simulink model "mechanical"  (R2019b)
settings: Solver=VariableStepAuto  StartTime=0.0  StopTime=10.0  RelTol=1e-3
undefined symbols (not defined in the file): B_hs, B_ks, beta, Cp, Cv, F_L, Fc, K_hs, K_ks, M, M_L, P_0, S_0, S_A, S_B, x0
libraries: simulink x2
settings Model: Creator=artof  LastModifiedBy=artof

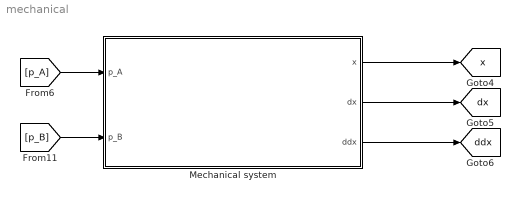
== system mechanical ==
  Mechanical system : Subsystem
  tag scope: ddx=global, dx=global, x=global
  wires:
  [p_A] -> Mechanical system/1(p_A)
  Mechanical system/1(x) -> [x]
  Mechanical system/2(dx) -> [dx]
  Mechanical system/3(ddx) -> [ddx]
  [p_B] -> Mechanical system/2(p_B)

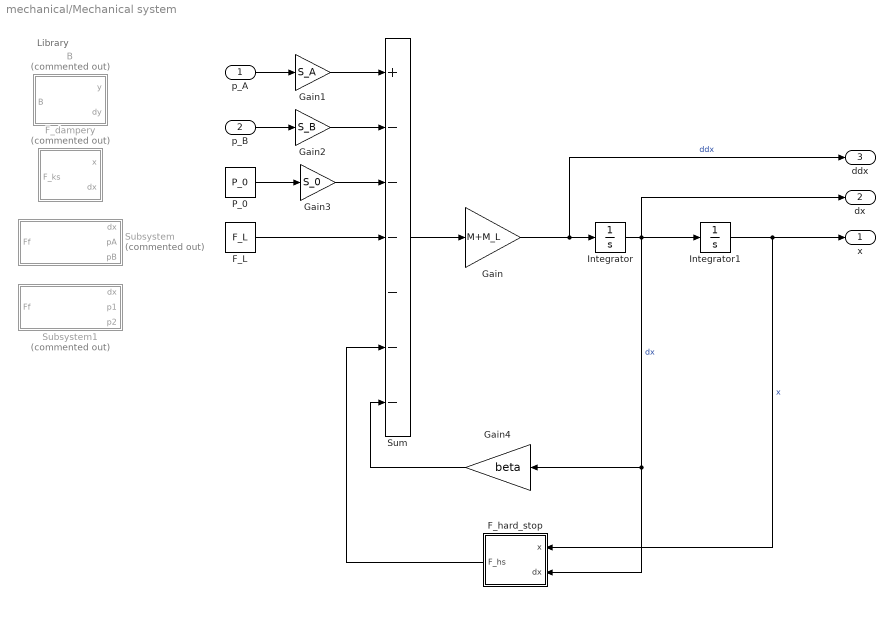
== system mechanical/Mechanical system ==
  note: Library
  p_A : Inport
  p_B : Inport  Port=2
  B : MATLAB Function  Commented=on  TreatAsAtomicUnit=on
  F_L : Constant  Value=F_L
  F_dampery : Subsystem  Commented=on
  F_hard_stop : Subsystem
  Gain : Gain  Gain=M+M_L
  Gain1 : Gain  Gain=S_A
  Gain2 : Gain  Gain=S_B
  Gain3 : Gain  Gain=S_0
  Gain4 : Gain  Gain=beta
  Integrator : Integrator
  Integrator1 : Integrator  InitialCondition=x0
  P_0 : Constant  Value=P_0
  Subsystem : Subsystem  Commented=on
  Subsystem1 : Subsystem  Commented=on
  Sum : Sum  Inputs=+------
  x : Outport
  dx : Outport  Port=2
  ddx : Outport  Port=3
  wires:
  p_A/1 -> Gain1/1
  Gain/1 -> ddx/1, Integrator/1  "ddx"
  Sum/1 -> Gain/1
  F_L/1 -> Sum/4
  P_0/1 -> Gain3/1
  Gain3/1 -> Sum/3
  Integrator/1 -> dx/1, F_hard_stop/2(dx), Gain4/1, Integrator1/1  "dx"
  Integrator1/1 -> x/1, F_hard_stop/1(x)  "x"
  p_B/1 -> Gain2/1
  Gain2/1 -> Sum/2
  F_hard_stop/1(F_hs) -> Sum/6
  Gain1/1 -> Sum/1
  Gain4/1 -> Sum/7

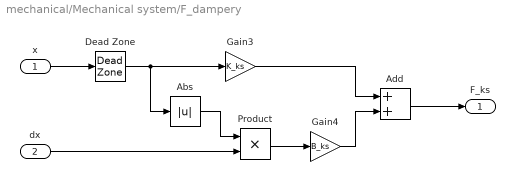
== system mechanical/Mechanical system/F_dampery ==
  x : Inport
  dx : Inport  Port=2
  Abs : Abs
  Add : Sum
  Dead Zone : DeadZone  LowerValue=0.02  UpperValue=0.180  SaturateOnIntegerOverflow=on
  Gain3 : Gain  Gain=K_ks
  Gain4 : Gain  Gain=B_ks
  Product : Product
  F_ks : Outport
  wires:
  Gain4/1 -> Add/2
  dx/1 -> Product/2
  Add/1 -> F_ks/1
  x/1 -> Dead Zone/1
  Gain3/1 -> Add/1
  Abs/1 -> Product/1
  Dead Zone/1 -> Abs/1, Gain3/1
  Product/1 -> Gain4/1

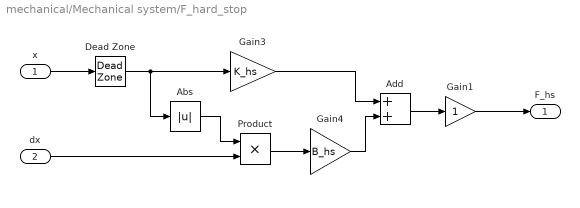
== system mechanical/Mechanical system/F_hard_stop ==
  x : Inport
  dx : Inport  Port=2
  Abs : Abs
  Add : Sum
  Dead Zone : DeadZone  LowerValue=0  UpperValue=L  SaturateOnIntegerOverflow=on
  Gain1 : Gain
  Gain3 : Gain  Gain=K_hs
  Gain4 : Gain  Gain=B_hs
  Product : Product
  F_hs : Outport
  wires:
  Product/1 -> Gain4/1
  Dead Zone/1 -> Gain3/1, Abs/1
  Abs/1 -> Product/1
  Gain3/1 -> Add/1
  x/1 -> Dead Zone/1
  Add/1 -> Gain1/1
  dx/1 -> Product/2
  Gain4/1 -> Add/2
  Gain1/1 -> F_hs/1

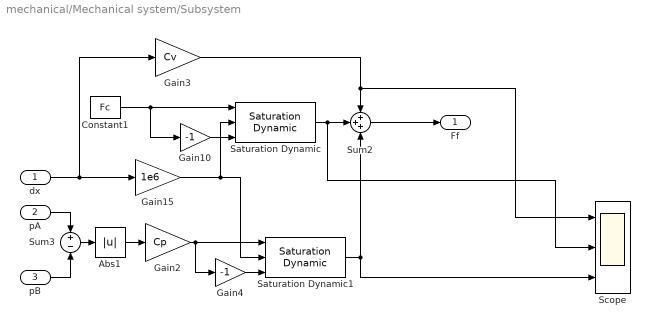
== system mechanical/Mechanical system/Subsystem ==
  dx : Inport
  pA : Inport  Port=2
  pB : Inport  Port=3
  Abs1 : Abs
  Constant1 : Constant  Value=Fc
  Gain10 : Gain  Gain=-1
  Gain15 : Gain  Gain=1e6
  Gain2 : Gain  Gain=Cp
  Gain3 : Gain  Gain=Cv
  Gain4 : Gain  Gain=-1
  Saturation Dynamic : simulink/Discontinuities/Saturation Dynamic  OutMin=[]  OutMax=[]  OutDataTypeStr=Inherit: Same as second input  OutDataType=sfix(16)  OutScaling=2^-10  DoSatur=off
  Saturation Dynamic1 : simulink/Discontinuities/Saturation Dynamic  OutMin=[]  OutMax=[]  OutDataTypeStr=Inherit: Same as second input  OutDataType=sfix(16)  OutScaling=2^-10  DoSatur=off
  Scope : Scope  NumInputPorts=3
  Sum2 : Sum  Inputs=+++
  Sum3 : Sum  Inputs=+|-
  Ff : Outport
  wires:
  Gain3/1 -> Scope/1, Sum2/1
  Gain2/1 -> Saturation Dynamic1/1, Gain4/1
  pA/1 -> Sum3/1
  dx/1 -> Gain3/1, Gain15/1
  pB/1 -> Sum3/2
  Saturation Dynamic1/1 -> Sum2/3, Scope/3
  Abs1/1 -> Gain2/1
  Sum2/1 -> Ff/1
  Gain15/1 -> Saturation Dynamic/2, Saturation Dynamic1/2
  Constant1/1 -> Saturation Dynamic/1, Gain10/1
  Gain4/1 -> Saturation Dynamic1/3
  Sum3/1 -> Abs1/1
  Gain10/1 -> Saturation Dynamic/3
  Saturation Dynamic/1 -> Scope/2, Sum2/2

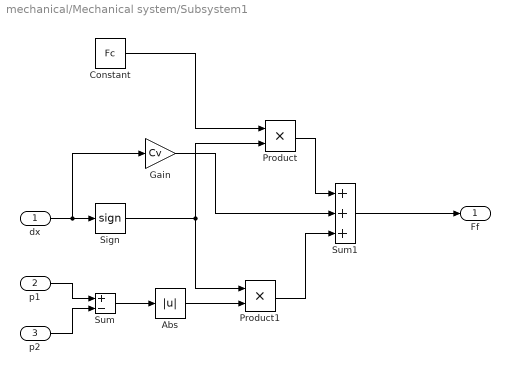
== system mechanical/Mechanical system/Subsystem1 ==
  dx : Inport
  p1 : Inport  Port=2
  p2 : Inport  Port=3
  Abs : Abs
  Constant : Constant  Value=Fc
  Gain : Gain  Gain=Cv
  Product : Product
  Product1 : Product
  Sign : Signum
  Sum : Sum  Inputs=+-
  Sum1 : Sum  Inputs=+++
  Ff : Outport
  wires:
  dx/1 -> Gain/1, Sign/1
  p2/1 -> Sum/2
  p1/1 -> Sum/1
  Sum/1 -> Abs/1
  Sign/1 -> Product/2, Product1/1
  Sum1/1 -> Ff/1
  Gain/1 -> Sum1/2
  Constant/1 -> Product/1
  Abs/1 -> Product1/2
  Product1/1 -> Sum1/3
  Product/1 -> Sum1/1

== matlab function mechanical/Mechanical system/B ==
  data: y input; B output; dy input
function B = fcn(y,dy)
%global b1 b2 b_max b_min
b_max   = 0.18;    %[m]
b_min   = 0.02;    %[m]
b1      = 100;    %[kg/s]
b2      = 100;    %[kg/s]   
if y > b_max && sign(dy) > 0
    B = b1;
elseif y < b_min && sign(dy) < 0 
    B = b2;
else
    B = 0;
end
end
